simulink library "Lib_Turbo_GearBox_TMATS"  (R2019b)
settings: Solver=ode45  StartTime=0.0  StopTime=10.0  RelTol=1e-3  EnableMultiTasking=on
Description:
  | Thomas Modules
settings Model: Creator=jwchapm2  LastModifiedBy=bhisma
settings DataIOCC: LimitDataPoints=on  SaveFormat=Array  ReturnWorkspaceOutputs=off
settings OptimizationCC: ExpressionDepthLimit=2147483647  LifeSpan=inf
settings DebuggingCC: UnderspecifiedInitializationDetection=Classic  MergeDetectMultiDrivingBlocksExec=none  SolverPrmCheckMsg=warning  StateNameClashWarn=warning  SFUnexpectedBacktrackingDiag=warning  SFNoUnconditionalDefaultTransitionDiag=warning  SFExecutionAtInitializationDiag=none  ArithmeticOperatorsInVariantConditions=warning
settings HardwareCC: ProdBitPerPointer=32  ProdBitPerSizeT=32  ProdBitPerPtrDiffT=32  ProdLargestAtomicFloat=None  ProdIntDivRoundTo=Undefined  ProdEndianess=Unspecified  ProdWordSize=32  ProdHWDeviceType=32-bit Generic
settings ModelReferenceCC: PropagateSignalLabelsOutOfModel=off
settings SFSimCC: SimUseLocalCustomCode=off  CustomCodeUndefinedFunction=UseInterfaceOnly
settings RTWCC: RTWUseLocalCustomCode=off
settings CodeAppCC: StateflowObjectComments=on
settings GRTTargetCC: TargetLangStandard=C89/C90 (ANSI)  GeneratePreprocessorConditionals=Disable all
settings ConfigComp: CovMetricSettings=dw  CovHtmlReporting=on  CovSaveCumulativeToWorkspaceVar=on  CovSaveSingleToWorkspaceVar=on  CovExternalEMLEnable=off

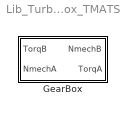
== system Lib_Turbo_GearBox_TMATS ==
  GearBox : Subsystem  mask(T-MATS: Gear Box Library Block){R_M=2, Eff_M=.99}
      mask prompts: R_M "R_M - Gear Ratio"; Eff_M "Eff_M - Efficiency (A to B)"
      mask help:
      | This block simulates the performance of a gear box using basic gear properties.
      |
      | Gear Ratio = NmechA/NmechB = TrqB/TrqA
      |
      | Where Nmech is the shaft speed and Trq is the shaft torque.
      mask Help: web(which('Turbo_TMATS_GBox.html'),'-helpbrowser')

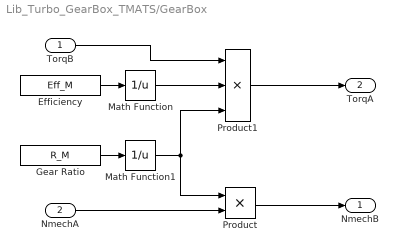
== system Lib_Turbo_GearBox_TMATS/GearBox ==
  TorqB : Inport
  NmechA : Inport  Port=2
  Efficiency : Constant  Value=Eff_M
  Gear Ratio : Constant  Value=R_M
  Math Function : Math  Operator=reciprocal  SaturateOnIntegerOverflow=on
  Math Function1 : Math  Operator=reciprocal  SaturateOnIntegerOverflow=on
  Product : Product  RndMeth=Zero
  Product1 : Product  Inputs=3  RndMeth=Zero
  NmechB : Outport
  TorqA : Outport  Port=2
  wires:
  Efficiency/1 -> Math Function/1
  TorqB/1 -> Product1/1
  Gear Ratio/1 -> Math Function1/1
  NmechA/1 -> Product/2
  Product1/1 -> TorqA/1
  Product/1 -> NmechB/1
  Math Function/1 -> Product1/2
  Math Function1/1 -> Product1/3, Product/1
